simulink model "UDPClent"  (R2018b)
settings: Solver=FixedStepDiscrete  StartTime=0.0  StopTime=inf  FixedStep=0.01  RelTol=1e-3
libraries: etargetslib x1, dspnetwork x1
settings Model: xpc_rtwmakecfg_data=_xpcnblib__xpcetherlib__xpcether8255xlib__xpcetherGbElib_  Creator=lenovo  LastModifiedBy=lenovo

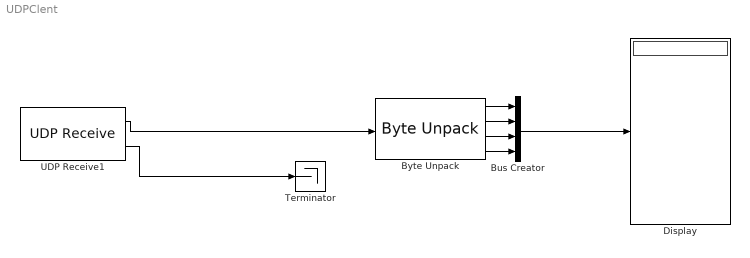
== system UDPClent ==
  Bus Creator : BusCreator  Inputs=4
  Byte Unpack : etargetslib/Byte Unpack  dimensions={[1],[1],[1],[1]}  datatypes={'double','double','double','double'}  byteAlign=4
  Display : Display
  Terminator : Terminator
  UDP Receive1 : dspnetwork/UDP Receive  localURL='0.0.0.0'  localPort=5432  remoteURL='127.0.0.1'  remotePort=-1  recvBufferSize=10240  dims=32  signalDatatype=uint8  isVarSize=off  showBlockingTime=off  blockingTime=0  sampletime=0.05  blockPlatform=[]
      settings: SourceProductName=DSP System Toolbox  SourceProductBaseCode=DS
  wires:
  UDP Receive1/1 -> Byte Unpack/1
  UDP Receive1/2 -> Terminator/1
  Byte Unpack/1 -> Bus Creator/1
  Byte Unpack/2 -> Bus Creator/2
  Byte Unpack/3 -> Bus Creator/3
  Byte Unpack/4 -> Bus Creator/4
  Bus Creator/1 -> Display/1
